simulink subsystem "NoSuspensionRearSSC"  (R2024b)
settings: Solver=VariableStepAuto  StartTime=0.0  StopTime=10.0  RelTol=1e-3
settings Model: ModifiedByFormat=The MathWorks, Inc.  Creator=The MathWorks, Inc.  LastModifiedBy=The MathWorks, Inc.
settings DebuggingCC: SubsystemReferenceDiagnosticForUnitTest=warning
settings RTWCC: GPUComputeCapability=3.5

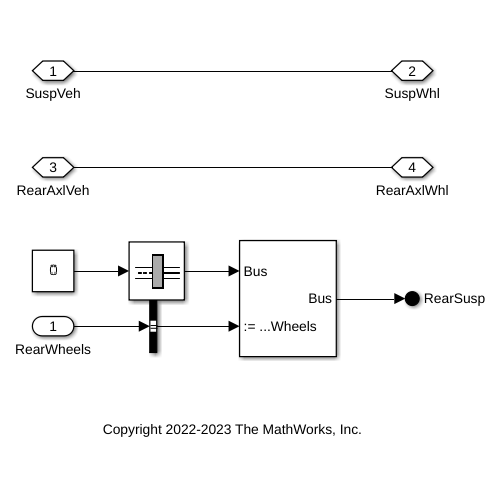
[thumbnail: Simulink's stored preview of the top-level diagram]
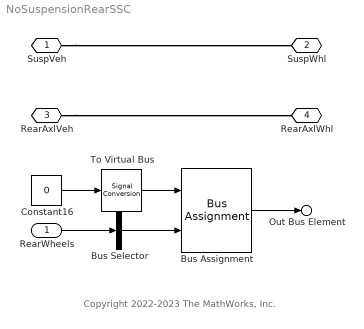
== system NoSuspensionRearSSC ==
  note: Copyright 2022-2023 The MathWorks, Inc.
  RearWheels : Inport
  Bus Assignment : BusAssignment  AssignedSignals=RearSuspWheel.Wheels
  Bus Selector : BusSelector  OutputSignals=Wheels  OutputAsBus=on
  Constant16 : Constant  Value=0  OutDataTypeStr=Bus: RearSuspBUS  SampleTime=Inf
  To Virtual Bus : SignalConversion  ConversionOutput=Virtual bus  OverrideOpt=off
  SuspVeh : PMIOPort  Side=Left
  SuspWhl : PMIOPort  Port=2  Side=Right
  RearAxlVeh : PMIOPort  Port=3  Side=Left
  RearAxlWhl : PMIOPort  Port=4  Side=Right
  Out Bus Element : Outport  PortName=RearSusp
  wires:
  RearWheels/1 -> Bus Selector/1
  Constant16/1 -> To Virtual Bus/1
  Bus Assignment/1 -> Out Bus Element/1
  To Virtual Bus/1 -> Bus Assignment/1
  Bus Selector/1 -> Bus Assignment/2
  connections:
  SuspVeh/RConn1 -- SuspWhl/RConn1
  RearAxlVeh/RConn1 -- RearAxlWhl/RConn1
